simulink model "smith_PID_tests1"  (R2018b)
settings: Solver=VariableStepAuto  StartTime=0.0  StopTime=25  RelTol=1e-3
libraries: simulink x1
settings Model: Creator=mmbio  LastModifiedBy=mmbio

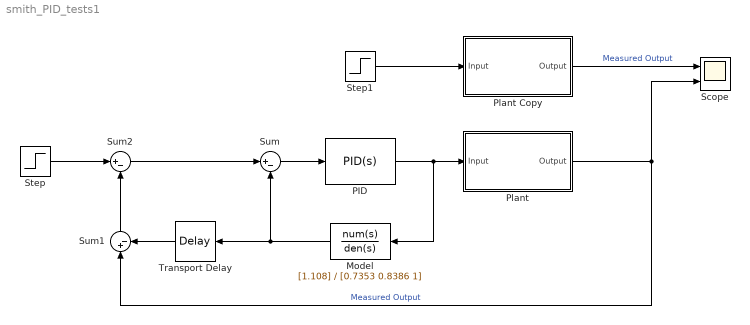
== system smith_PID_tests1 ==
  Model : TransferFcn  Numerator=[1.108]  Denominator=[0.7353 0.8386 1]
  PID : simulink/Continuous/PID Controller  Controller=PID  Form=Parallel  TimeDomain=Continuous-time  SampleTime=-1  IntegratorMethod=Forward Euler  FilterMethod=Forward Euler  ControllerParametersSource=internal  P=0.770971991004443  I=0.690345188253394  D=0.150628440266954  UseFilter=on  N=132.702618316638  TunerSelectOption=Transfer Function Based (PID Tuner App)  InitialConditionSource=internal  InitialConditionForIntegrator=0  InitialConditionForFilter=0  DifferentiatorICPrevScaledInput=0  ExternalReset=none  TrackingMode=off  Kt=1  LimitOutput=off  UpperSaturationLimit=inf  LowerSaturationLimit=-inf  LinearizeAsGain=on  AntiWindupMode=none  Kb=1  POutMin=[]  POutMax=[]  IOutMin=[]  IOutMax=[]  DOutMin=[]  DOutMax=[]  NOutMin=[]  NOutMax=[]  SumOutMin=[]  SumOutMax=[]  SaturationOutMin=[]  SaturationOutMax=[]  PParamMin=[]  PParamMax=[]  IParamMin=[]  IParamMax=[]  DParamMin=[]  DParamMax=[]  NParamMin=[]  NParamMax=[]  KbParamMin=[]  KbParamMax=[]  KtParamMin=[]  KtParamMax=[]  KbOutMin=[]  KbOutMax=[]  KtOutMin=[]  KtOutMax=[]  IntegratorOutMin=[]  IntegratorOutMax=[]  FilterOutMin=[]  FilterOutMax=[]  SumI1OutMin=[]  SumI1OutMax=[]  SumI2OutMin=[]  SumI2OutMax=[]  SumI3OutMin=[]  SumI3OutMax=[]  SumI4OutMin=[]  SumI4OutMax=[]  SumDOutMin=[]  SumDOutMax=[]  DifferentiatorOutMin=[]  DifferentiatorOutMax=[]  FilterDiffOutCoefMin=[]  FilterDiffOutCoefMax=[]  ReciprocalOutMin=[]  ReciprocalOutMax=[]  SumDenOutMin=[]  SumDenOutMax=[]  SumNumOutMin=[]  SumNumOutMax=[]  DivideOutMin=[]  DivideOutMax=[]  IntegratorContinuousStateAttributes=''  IntegratorStateMustResolveToSignalObject=off  IntegratorRTWStateStorageClass=Auto  FilterContinuousStateAttributes=''  FilterStateMustResolveToSignalObject=off  FilterRTWStateStorageClass=Auto  ParallelPVariant=InternalParameters  IdealPVariant=Disabled  IVariant=InternalParameters  DVariant=InternalParameters  IntegratorVariant=Continuous  SatVariant=Disabled  AWVariant=Passthrough  PCopyVariant=Disabled  TRVariant=Disabled  FdbkBlocksVariant=Forward  IdealPFdbkVariant=Disabled  SatFdbkVariant=Disabled  DerivativeFilterVariant=ContFilter  NVariant=InternalParameters  NCopyVariant=Disabled  FilterICVariant=InternalICsFilter  IntegratorICVariant=InternalICs  ExternalResetVariant=Disabled  TRSumVariant=Passthrough  SumFdbkVariant=Disabled  SumVariant=Sum_PID
  Plant : Subsystem
  Plant Copy : Subsystem
  Scope : Scope  NumInputPorts=2
  Step : Step  After=1.108  SampleTime=0
  Step1 : Step  SampleTime=0
  Sum : Sum  Inputs=|+-
  Sum1 : Sum  Inputs=|+-
  Sum2 : Sum  Inputs=|+-
  Transport Delay : TransportDelay  DelayTime=0.45
  wires:
  Step/1 -> Sum2/1
  Transport Delay/1 -> Sum1/2
  Plant/1(Output) -> Scope/2, Sum1/1  "Measured Output"
  Sum2/1 -> Sum/1
  Plant Copy/1(Output) -> Scope/1  "Measured Output"
  Step1/1 -> Plant Copy/1(Input)
  Sum1/1 -> Sum2/2
  Model/1 -> Transport Delay/1, Sum/2
  PID/1 -> Model/1, Plant/1(Input)
  Sum/1 -> PID/1

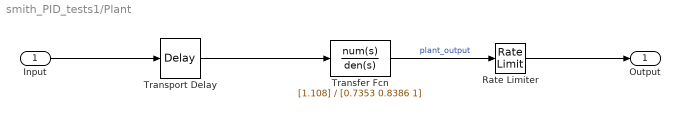
== system smith_PID_tests1/Plant ==
  Input : Inport
  Rate Limiter : RateLimiter  RisingSlewLimit=0.657875  FallingSlewLimit=-0.657875  SampleTimeMode=inherited
  Transfer Fcn : TransferFcn  Numerator=[1.108]  Denominator=[0.7353 0.8386 1]
  Transport Delay : TransportDelay  DelayTime=0.45
  Output : Outport
  wires:
  Input/1 -> Transport Delay/1
  Transfer Fcn/1 -> Rate Limiter/1  "plant_output"
  Transport Delay/1 -> Transfer Fcn/1
  Rate Limiter/1 -> Output/1

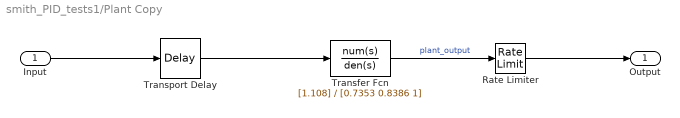
== system smith_PID_tests1/Plant Copy ==
  Input : Inport
  Rate Limiter : RateLimiter  RisingSlewLimit=0.657875  FallingSlewLimit=-0.657875  SampleTimeMode=inherited
  Transfer Fcn : TransferFcn  Numerator=[1.108]  Denominator=[0.7353 0.8386 1]
  Transport Delay : TransportDelay  DelayTime=0.45
  Output : Outport
  wires:
  Input/1 -> Transport Delay/1
  Transfer Fcn/1 -> Rate Limiter/1  "plant_output"
  Transport Delay/1 -> Transfer Fcn/1
  Rate Limiter/1 -> Output/1
